simulink subsystem "NLMPCController"  (R2022b)
settings: Solver=VariableStepAuto  StartTime=0.0  StopTime=10.0  RelTol=1e-3
undefined symbols (not defined in the file): Cf, Cr, egoVehDyn, Iz, lf, lr, m, tau, Ts, v_set
libraries: sharedTrackingLibrary x1, mpclib x1
settings Model: Creator=The MathWorks, Inc.  LastModifiedBy=The MathWorks, Inc.
settings SolverCC: MaxZcPerStep=1
settings ModelReferenceCC: EnableRefExpFcnMdlSchedulingChecks=on
settings RTWCC: DLArmComputeVersion=19.05

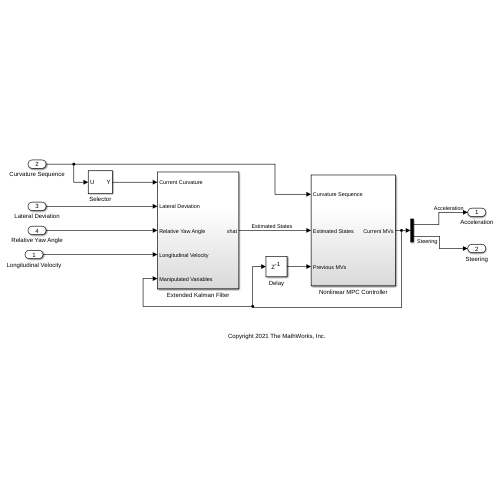
[thumbnail: Simulink's stored preview of the top-level diagram]
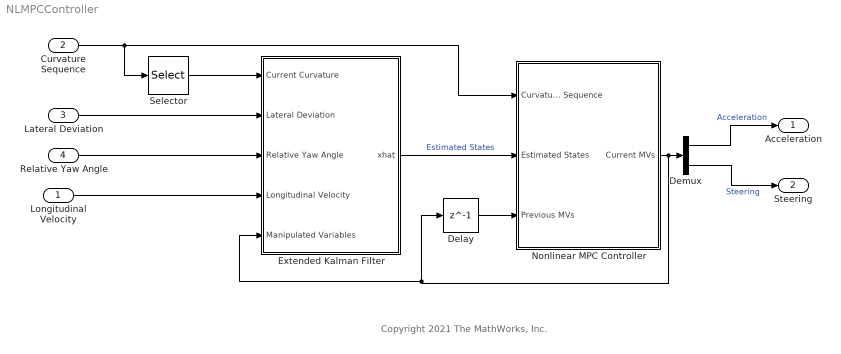
== system NLMPCController ==
  note: Copyright 2021 The MathWorks, Inc.
  Longitudinal Velocity : Inport
  Curvature Sequence : Inport  Port=2
  Lateral Deviation : Inport  Port=3
  Relative Yaw Angle : Inport  Port=4
  Delay : Delay  DelayLength=1  InitialCondition=[0.2 0.3]
  Demux : Demux  Outputs=2
  Extended Kalman Filter : Subsystem
  Nonlinear MPC Controller : Subsystem
  Selector : Selector  InputPortWidth=predictionHorizon  IndexOptions=Index vector (dialog)  Indices=1  OutputSizes=1
  Acceleration : Outport  VectorParamsAs1DForOutWhenUnconnected=off
  Steering : Outport  Port=2  VectorParamsAs1DForOutWhenUnconnected=off
  wires:
  Extended Kalman Filter/1(xhat) -> Nonlinear MPC Controller/2(Estimated States)  "Estimated States"
  Nonlinear MPC Controller/1(Current MVs) -> Demux/1, Delay/1, Extended Kalman Filter/5(Manipulated Variables)
  Lateral Deviation/1 -> Extended Kalman Filter/2(Lateral Deviation)
  Longitudinal Velocity/1 -> Extended Kalman Filter/4(Longitudinal Velocity)
  Delay/1 -> Nonlinear MPC Controller/3(Previous MVs)
  Relative Yaw Angle/1 -> Extended Kalman Filter/3(Relative Yaw Angle)
  Demux/2 -> Steering/1  "Steering"
  Demux/1 -> Acceleration/1  "Acceleration"
  Curvature Sequence/1 -> Selector/1, Nonlinear MPC Controller/1(Curvature Sequence)
  Selector/1 -> Extended Kalman Filter/1(Current Curvature)

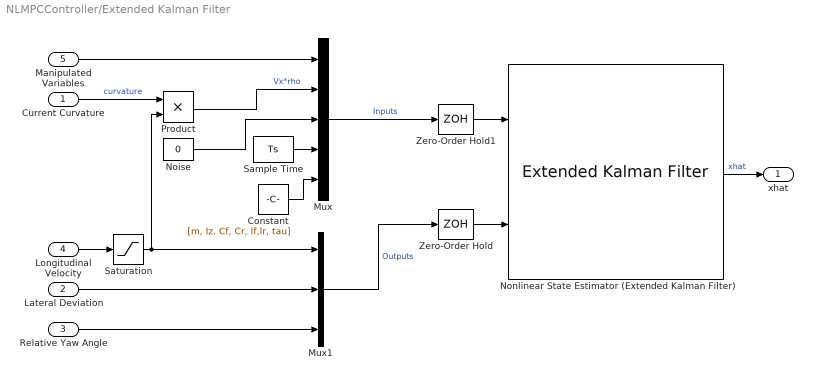
== system NLMPCController/Extended Kalman Filter ==
  Current Curvature : Inport
  Lateral Deviation : Inport  Port=2
  Relative Yaw Angle : Inport  Port=3
  Longitudinal Velocity : Inport  Port=4
  Manipulated Variables : Inport  Port=5
  Constant : Constant  Value=[m, Iz, Cf, Cr, lf,lr, tau]
  Mux : Mux  Inputs=5
  Mux1 : Mux  Inputs=3
  Noise : Constant  Value=0
  Nonlinear State Estimator (Extended Kalman Filter) : sharedTrackingLibrary/Extended Kalman Filter  StateTransitionFcn=helperEKFStateFcn  HasStateTransitionJacobianFcn=off  HasAdditiveProcessNoise=Additive  ProcessNoise=1e-4*eye(7)  HasTimeVaryingProcessNoise=off  HasStateTransitionFcnExtraArgument=1  InitialState=[0 0 egoVehDyn.VLong0 0 0 0 0]'  InitialStateCovariance=1e-4*eye(7)  MeasurementFcn1=helperEKFMeasFcn  HasMeasurementJacobianFcn1=off  HasMeasurementEnablePort1=off  HasAdditiveMeasurementNoise1=Additive  MeasurementNoise1=1e-4*eye(3)  HasTimeVaryingMeasurementNoise1=off  HasMeasurementFcnExtraArgument1=0  HasMeasurementWrapping1=off  MeasurementFcn2=myMeasurementFcn  HasMeasurementJacobianFcn2=off  HasMeasurementEnablePort2=off  HasAdditiveMeasurementNoise2=Additive  MeasurementNoise2=1  HasTimeVaryingMeasurementNoise2=off  HasMeasurementFcnExtraArgument2=0  HasMeasurementWrapping2=off  MeasurementFcn3=myMeasurementFcn  HasMeasurementJacobianFcn3=off  HasMeasurementEnablePort3=off  HasAdditiveMeasurementNoise3=Additive  MeasurementNoise3=1  HasTimeVaryingMeasurementNoise3=off  HasMeasurementFcnExtraArgument3=0  HasMeasurementWrapping3=off  MeasurementFcn4=myMeasurementFcn  HasMeasurementJacobianFcn4=off  HasMeasurementEnablePort4=off  HasAdditiveMeasurementNoise4=Additive  MeasurementNoise4=1  HasTimeVaryingMeasurementNoise4=off  HasMeasurementFcnExtraArgument4=0  HasMeasurementWrapping4=off  MeasurementFcn5=myMeasurementFcn  HasMeasurementJacobianFcn5=off  HasMeasurementEnablePort5=off  HasAdditiveMeasurementNoise5=Additive  MeasurementNoise5=1  HasTimeVaryingMeasurementNoise5=off  HasMeasurementFcnExtraArgument5=0  HasMeasurementWrapping5=off  EnableMultirate=off  StateTransitionFcnSampleTime=1  MeasurementFcn1SampleTime=1  MeasurementFcn2SampleTime=1  MeasurementFcn3SampleTime=1  MeasurementFcn4SampleTime=1  MeasurementFcn5SampleTime=1  UseCurrentEstimator=on  OutputStateCovariance=off  DataType=double  SampleTime=Ts  NumberOfMeasurements=1
  Product : Product
  Sample Time : Constant  Value=Ts
  Saturation : Saturate  UpperLimit=inf  LowerLimit=0.2
  Zero-Order Hold : ZeroOrderHold  SampleTime=Ts
  Zero-Order Hold1 : ZeroOrderHold  SampleTime=Ts
  xhat : Outport  VectorParamsAs1DForOutWhenUnconnected=off
  wires:
  Saturation/1 -> Mux1/1, Product/2
  Longitudinal Velocity/1 -> Saturation/1
  Constant/1 -> Mux/5
  Zero-Order Hold1/1 -> Nonlinear State Estimator (Extended Kalman Filter)/1
  Mux/1 -> Zero-Order Hold1/1  "Inputs"
  Product/1 -> Mux/2  "Vx*rho"
  Current Curvature/1 -> Product/1  "curvature"
  Relative Yaw Angle/1 -> Mux1/3
  Lateral Deviation/1 -> Mux1/2
  Mux1/1 -> Zero-Order Hold/1  "Outputs"
  Nonlinear State Estimator (Extended Kalman Filter)/1 -> xhat/1  "xhat"
  Sample Time/1 -> Mux/4
  Manipulated Variables/1 -> Mux/1
  Zero-Order Hold/1 -> Nonlinear State Estimator (Extended Kalman Filter)/2
  Noise/1 -> Mux/3

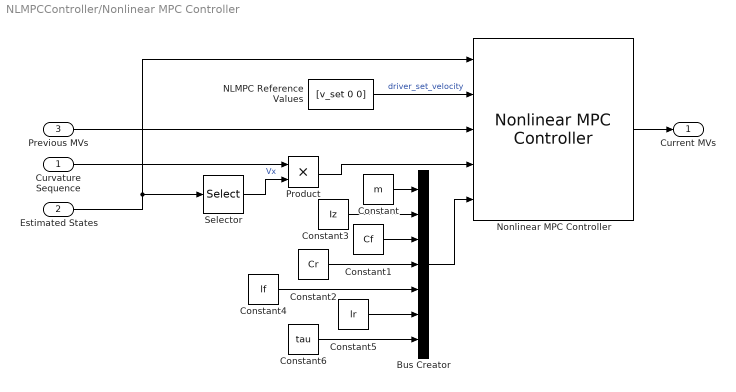
== system NLMPCController/Nonlinear MPC Controller ==
  Curvature Sequence : Inport
  Estimated States : Inport  Port=2
  Previous MVs : Inport  Port=3
  Bus Creator : BusCreator  Inputs=7  OutDataTypeStr=Bus: paramsBusObject  NonVirtualBus=on
      settings: InheritFromInputs=off
  Constant : Constant  Value=m
  Constant1 : Constant  Value=Cf
  Constant2 : Constant  Value=Cr
  Constant3 : Constant  Value=Iz
  Constant4 : Constant  Value=lf
  Constant5 : Constant  Value=lr
  Constant6 : Constant  Value=tau
  NLMPC Reference Values : Constant  Value=[v_set 0 0]  VectorParams1D=off
  Nonlinear MPC Controller : mpclib/Nonlinear MPC Controller  SCDEnableBlockLinearizationSpecification=on  nlmpcobj=nlobj  UseObjectTs=off  TsControl=NLMPCTs  UseMEX=off  md_enabled=on  mvtarget_enabled=off  param_enabled=on  cost_enabled=off  mvseq_enabled=off  stateseq_enabled=off  ovseq_enabled=off  slack_enabled=off  status_enabled=off  ov_min=off  ov_max=off  mv_min=off  mv_max=off  mvrate_min=off  mvrate_max=off  state_min=off  state_max=off  ov_weight=off  mv_weight=off  mvrate_weight=off  ecr_weight=off  nlp_initialize=off
  Product : Product
  Selector : Selector  InputPortWidth=7  IndexOptions=Index vector (dialog)  Indices=[3]  OutputSizes=1
  Current MVs : Outport  VectorParamsAs1DForOutWhenUnconnected=off
  wires:
  Constant6/1 -> Bus Creator/7
  Constant5/1 -> Bus Creator/6
  Constant4/1 -> Bus Creator/5
  Constant2/1 -> Bus Creator/4
  Constant1/1 -> Bus Creator/3
  Constant3/1 -> Bus Creator/2
  Constant/1 -> Bus Creator/1
  Bus Creator/1 -> Nonlinear MPC Controller/5
  Product/1 -> Nonlinear MPC Controller/4
  Curvature Sequence/1 -> Product/1
  Selector/1 -> Product/2  "Vx"
  Nonlinear MPC Controller/1 -> Current MVs/1
  Estimated States/1 -> Selector/1, Nonlinear MPC Controller/1
  NLMPC Reference Values/1 -> Nonlinear MPC Controller/2  "driver_set_velocity"
  Previous MVs/1 -> Nonlinear MPC Controller/3
